simulink model "train_model_la_nika"  (R2021b)
settings: Solver=VariableStepAuto  StartTime=0.0  StopTime=10.0  RelTol=1e-3
undefined symbols (not defined in the file): g, nx, ny
settings Model: Creator=Acer  LastModifiedBy=Acer

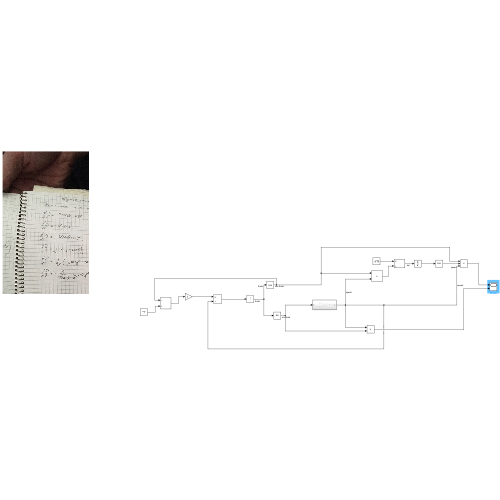
[thumbnail: Simulink's stored preview of the top-level diagram]
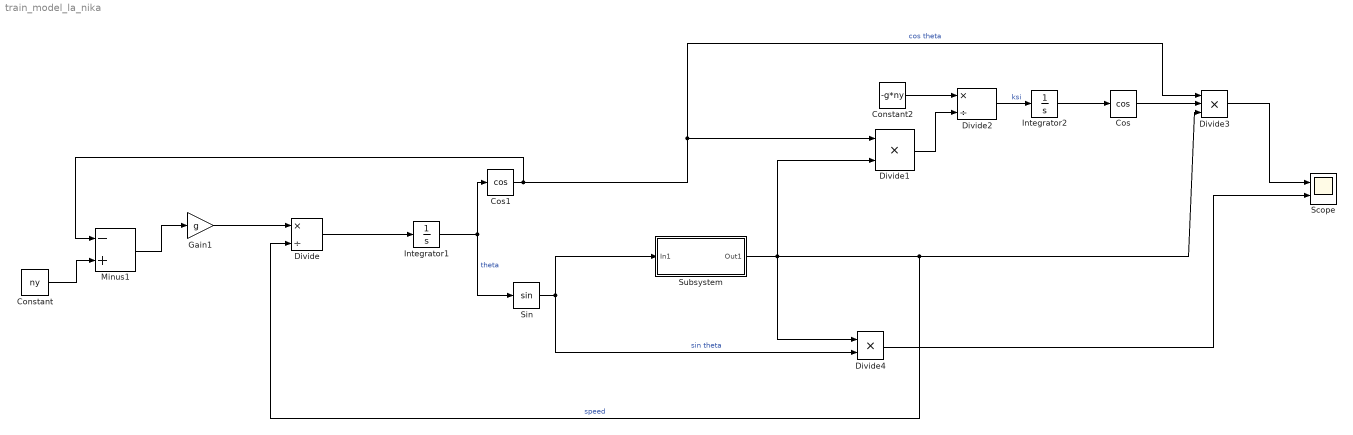
== system train_model_la_nika ==
  Constant : Constant  Value=ny
  Constant2 : Constant  Value=-g*ny
  Cos : Trigonometry  Operator=cos
  Cos1 : Trigonometry  Operator=cos
  Divide : Product  Inputs=*/
  Divide1 : Product  Inputs=**
  Divide2 : Product  Inputs=*/
  Divide3 : Product  Inputs=***
  Divide4 : Product  Inputs=**
  Gain1 : Gain  Gain=g
  Integrator1 : Integrator
  Integrator2 : Integrator
  Minus1 : Sum  Inputs=-+
  Scope : Scope  NumInputPorts=2
  Sin : Trigonometry
  Subsystem : Subsystem
  wires:
  Integrator1/1 -> Sin/1, Cos1/1  "theta"
  Sin/1 -> Subsystem/1(In1), Divide4/2  "sin theta"
  Minus1/1 -> Gain1/1
  Subsystem/1(Out1) -> Divide4/1, Divide/2, Divide3/3, Divide1/2  "speed"
  Divide/1 -> Integrator1/1
  Constant2/1 -> Divide2/1
  Divide1/1 -> Divide2/2
  Divide2/1 -> Integrator2/1  "ksi"
  Integrator2/1 -> Cos/1
  Cos/1 -> Divide3/2
  Divide3/1 -> Scope/1
  Divide4/1 -> Scope/2
  Gain1/1 -> Divide/1
  Constant/1 -> Minus1/2
  Cos1/1 -> Divide3/1, Divide1/1, Minus1/1  "cos theta"

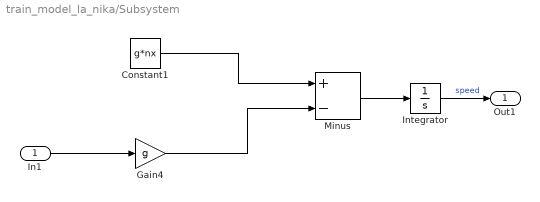
== system train_model_la_nika/Subsystem ==
  In1 : Inport
  Constant1 : Constant  Value=g*nx
  Gain4 : Gain  Gain=g
  Integrator : Integrator  InitialCondition=100
  Minus : Sum  Inputs=+-
  Out1 : Outport
  wires:
  Constant1/1 -> Minus/1
  Minus/1 -> Integrator/1
  Gain4/1 -> Minus/2
  Integrator/1 -> Out1/1  "speed"
  In1/1 -> Gain4/1
